simulink model "Accelerator_Pedal_Position_Sensor"  (R2018a)
settings: Solver=VariableStepAuto  StartTime=0.0  StopTime=10.0  RelTol=1e-3
settings Model: Creator=Choaib ELMADI  LastModifiedBy=Choaib ELMADI
settings DataIOCC: LoadExternalInput=on

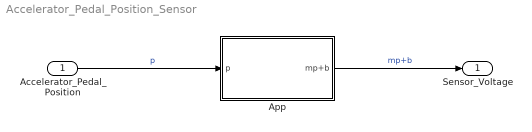
== system Accelerator_Pedal_Position_Sensor ==
  Accelerator_Pedal_Position : Inport
  App : Subsystem
  Sensor_Voltage : Outport
  wires:
  Accelerator_Pedal_Position/1 -> App/1(p)  "p"
  App/1(mp+b) -> Sensor_Voltage/1  "mp+b"

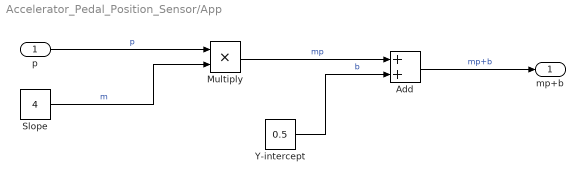
== system Accelerator_Pedal_Position_Sensor/App ==
  p : Inport
  Add : Sum
  Multiply : Product
  Slope : Constant  Value=4
  Y-intercept : Constant  Value=0.5
  mp+b : Outport
  wires:
  Slope/1 -> Multiply/2  "m"
  Multiply/1 -> Add/1  "mp"
  Y-intercept/1 -> Add/2  "b"
  Add/1 -> mp+b/1  "mp+b"
  p/1 -> Multiply/1  "p"
